simulink model "sim_qpOases_uncondensed"  (R2020b)
settings: Solver=FixedStepAuto  StartTime=0.0  StopTime=T_sim  FixedStep=dt  RelTol=1e-3
undefined symbols (not defined in the file): A_alpha1, A_init, A_TEC, Adyn_e, Adyn_t, b_alpha1, b_dyn, b_TEC, C, dt, H_e, H_t, L, lambda_beta, lb, m, N, NOISE, noise_bound_cl, nu, p, Sy_e, Sy_t, T_Track, T_Track2, T_Track3, ub, x0, y_T1, y_T2, y_T3, y_T4
libraries: simulink x5
settings Model: Creator=Fabian  LastModifiedBy=Fabian

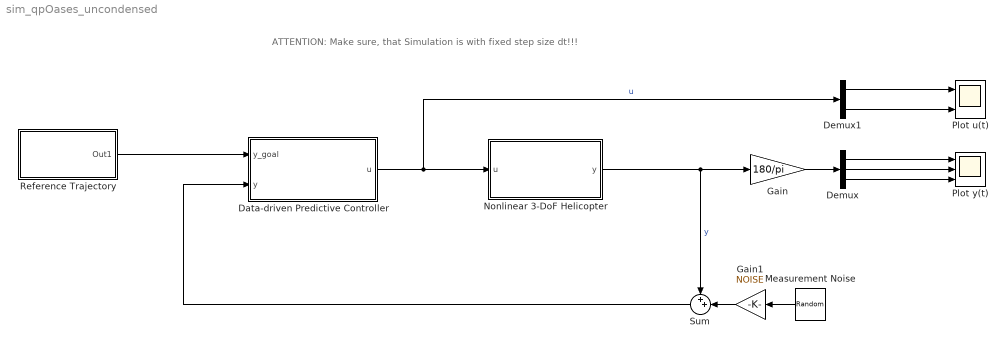
== system sim_qpOases_uncondensed ==
  note: ATTENTION: Make sure, that Simulation is with fixed step size dt!!!
  Data-driven Predictive Controller : Subsystem
  Demux : Demux  Outputs=3
  Demux1 : Demux  Outputs=2
  Gain : Gain  Gain=180/pi
  Gain1 : Gain  Gain=NOISE
  Measurement Noise : UniformRandomNumber  Minimum=-noise_bound_cl  Maximum=noise_bound_cl  Seed=[3;4;5]  SampleTime=dt
  Nonlinear 3-DoF Helicopter : Subsystem
  Plot u(t) : Scope  NumInputPorts=2
  Plot y(t) : Scope  NumInputPorts=3
  Reference Trajectory : Subsystem
  Sum : Sum  Inputs=++|
  wires:
  Data-driven Predictive Controller/1(u) -> Demux1/1, Nonlinear 3-DoF Helicopter/1(u)  "u"
  Measurement Noise/1 -> Gain1/1
  Nonlinear 3-DoF Helicopter/1(y) -> Gain/1, Sum/1  "y"
  Gain1/1 -> Sum/2
  Gain/1 -> Demux/1
  Sum/1 -> Data-driven Predictive Controller/2(y)
  Demux/2 -> Plot y(t)/2
  Demux/1 -> Plot y(t)/1
  Demux/3 -> Plot y(t)/3
  Reference Trajectory/1(Out1) -> Data-driven Predictive Controller/1(y_goal)
  Demux1/1 -> Plot u(t)/1
  Demux1/2 -> Plot u(t)/2

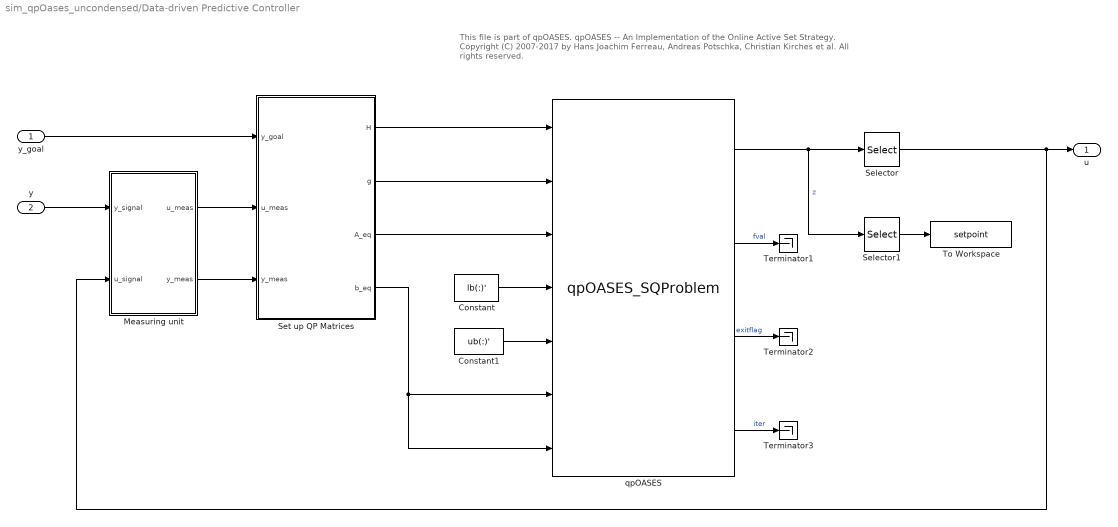
== system sim_qpOases_uncondensed/Data-driven Predictive Controller ==
  note: This file is part of qpOASES.
      |
      | qpOASES -- An Implementation of the Online Active Set Strategy.
      | Copyright (C) 2007-2017 by Hans Joachim Ferreau, Andreas Potschka, Christian Kirches et al.
      | All rights reserved.
  y_goal : Inport
  y : Inport  Port=2
  Constant : Constant  Value=lb(:)'
  Constant1 : Constant  Value=ub(:)'
  Measuring unit : Subsystem
  Selector : Selector  InputPortWidth=N-L+1+m*L+p*L+m+p+p*L+1  IndexOptions=Index vector (dialog)  Indices=N-L+1+m*nu+1:N-L+1+m*nu+m  OutputSizes=1
  Selector1 : Selector  InputPortWidth=N-L+1+m*L+p*L+m+p+p*L+1  IndexOptions=Index vector (dialog)  Indices=N-L+1+m*L+p*L+m+1:N-L+1+m*L+p*L+m+p  OutputSizes=1
  Set up QP Matrices : MATLAB Function  TreatAsAtomicUnit=on
  Terminator1 : Terminator
  Terminator2 : Terminator
  Terminator3 : Terminator
  To Workspace : ToWorkspace  VariableName=setpoint  SaveFormat=Timeseries  SampleTime=-1
  qpOASES : S-Function  FunctionName=qpOASES_SQProblem  SFunctionDeploymentMode=off  EnableBusSupport=off
  u : Outport
  wires:
  y/1 -> Measuring unit/1(y_signal)
  Measuring unit/1(u_meas) -> Set up QP Matrices/2(u_meas)
  Measuring unit/2(y_meas) -> Set up QP Matrices/3(y_meas)
  y_goal/1 -> Set up QP Matrices/1(y_goal)
  Selector/1 -> u/1, Measuring unit/2(u_signal)
  Set up QP Matrices/1(H) -> qpOASES/1
  qpOASES/1 -> Selector1/1, Selector/1  "z"
  Constant/1 -> qpOASES/4
  Set up QP Matrices/4(b_eq) -> qpOASES/6, qpOASES/7
  qpOASES/4 -> Terminator3/1  "iter"
  qpOASES/3 -> Terminator2/1  "exitflag"
  qpOASES/2 -> Terminator1/1  "fval"
  Set up QP Matrices/2(g) -> qpOASES/2
  Set up QP Matrices/3(A_eq) -> qpOASES/3
  Constant1/1 -> qpOASES/5
  Selector1/1 -> To Workspace/1

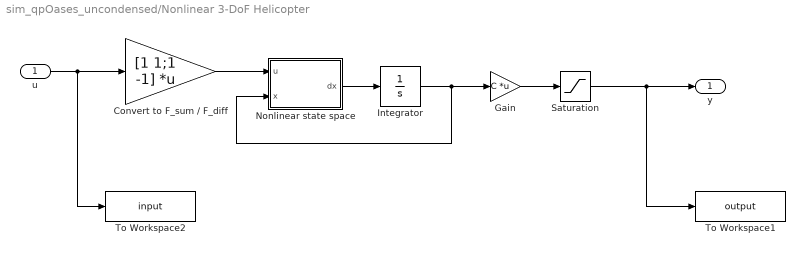
== system sim_qpOases_uncondensed/Nonlinear 3-DoF Helicopter ==
  u : Inport
  Convert to F_sum / F_diff : Gain  Gain=[1 1;1 -1]  Multiplication=Matrix(K*u)
  Gain : Gain  Gain=C  Multiplication=Matrix(K*u)
  Integrator : Integrator  InitialCondition=x0
  Nonlinear state space : MATLAB Function  TreatAsAtomicUnit=on
  Saturation : Saturate  UpperLimit=[inf; 33*pi/180; 90*pi/180]  LowerLimit=[-inf; -33*pi/180; -90*pi/180]
  To Workspace1 : ToWorkspace  VariableName=output  SaveFormat=Timeseries  SampleTime=-1
  To Workspace2 : ToWorkspace  VariableName=input  SaveFormat=Timeseries  SampleTime=-1
  y : Outport
  wires:
  Nonlinear state space/1(dx) -> Integrator/1
  Integrator/1 -> Nonlinear state space/2(x), Gain/1
  u/1 -> To Workspace2/1, Convert to F_sum / F_diff/1
  Convert to F_sum / F_diff/1 -> Nonlinear state space/1(u)
  Gain/1 -> Saturation/1
  Saturation/1 -> To Workspace1/1, y/1

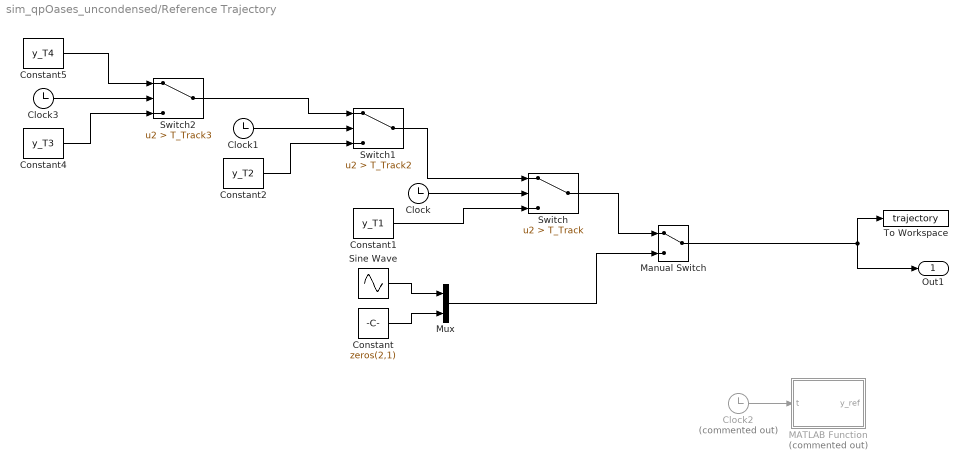
== system sim_qpOases_uncondensed/Reference Trajectory ==
  Clock : Clock
  Clock1 : Clock
  Clock2 : Clock  Commented=on
  Clock3 : Clock
  Constant : Constant  Value=zeros(2,1)
  Constant1 : Constant  Value=y_T1
  Constant2 : Constant  Value=y_T2
  Constant4 : Constant  Value=y_T3
  Constant5 : Constant  Value=y_T4
  MATLAB Function : MATLAB Function  Commented=on  TreatAsAtomicUnit=on
  Manual Switch : ManualSwitch
  Mux : Mux  Inputs=2
  Sine Wave : Sin  Amplitude=45*pi/180  Frequency=2*pi*1/25  Phase=-5*2*pi*1/25  SampleTime=0
  Switch : Switch  Criteria=u2 > Threshold  Threshold=T_Track
  Switch1 : Switch  Criteria=u2 > Threshold  Threshold=T_Track2
  Switch2 : Switch  Criteria=u2 > Threshold  Threshold=T_Track3
  To Workspace : ToWorkspace  VariableName=trajectory  SaveFormat=Timeseries  SampleTime=-1
  Out1 : Outport
  wires:
  Manual Switch/1 -> Out1/1, To Workspace/1
  Switch2/1 -> Switch1/1
  Mux/1 -> Manual Switch/2
  Constant2/1 -> Switch1/3
  Clock1/1 -> Switch1/2
  Clock/1 -> Switch/2
  Sine Wave/1 -> Mux/1
  Constant/1 -> Mux/2
  Switch/1 -> Manual Switch/1
  Switch1/1 -> Switch/1
  Constant1/1 -> Switch/3
  Clock2/1 -> MATLAB Function/1(t)
  Clock3/1 -> Switch2/2
  Constant5/1 -> Switch2/1
  Constant4/1 -> Switch2/3

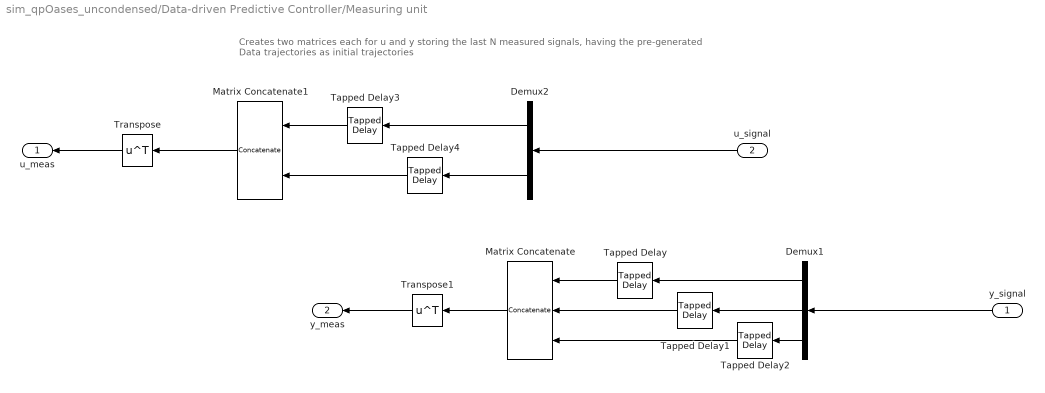
== system sim_qpOases_uncondensed/Data-driven Predictive Controller/Measuring unit ==
  note: Creates two matrices each for u and y storing the last N measured signals,
      | having the pre-generated Data trajectories as initial trajectories
  y_signal : Inport
  u_signal : Inport  Port=2
  Demux1 : Demux  Outputs=3
  Demux2 : Demux  Outputs=2
  Matrix Concatenate : Concatenate  NumInputs=3  Mode=Multidimensional array  ConcatenateDimension=2
  Matrix Concatenate1 : Concatenate  Mode=Multidimensional array  ConcatenateDimension=2
  Tapped Delay : simulink/Discrete/Tapped Delay  vinit=x0(1)*ones(nu,1)  samptime=-1  NumDelays=nu  DelayOrder=Oldest  includeCurrent=off
  Tapped Delay1 : simulink/Discrete/Tapped Delay  vinit=x0(3)*ones(nu,1)  samptime=-1  NumDelays=nu  DelayOrder=Oldest  includeCurrent=off
  Tapped Delay2 : simulink/Discrete/Tapped Delay  vinit=x0(5)*ones(nu,1)  samptime=-1  NumDelays=nu  DelayOrder=Oldest  includeCurrent=off
  Tapped Delay3 : simulink/Discrete/Tapped Delay  vinit=0  samptime=-1  NumDelays=nu  DelayOrder=Oldest  includeCurrent=off
  Tapped Delay4 : simulink/Discrete/Tapped Delay  vinit=0  samptime=-1  NumDelays=nu  DelayOrder=Oldest  includeCurrent=off
  Transpose : Math  Operator=transpose  SaturateOnIntegerOverflow=on
  Transpose1 : Math  Operator=transpose  SaturateOnIntegerOverflow=on
  u_meas : Outport
  y_meas : Outport  Port=2
  wires:
  Demux2/2 -> Tapped Delay4/1
  Demux2/1 -> Tapped Delay3/1
  Tapped Delay3/1 -> Matrix Concatenate1/1
  Demux1/1 -> Tapped Delay/1
  Demux1/2 -> Tapped Delay1/1
  Tapped Delay4/1 -> Matrix Concatenate1/2
  Demux1/3 -> Tapped Delay2/1
  Tapped Delay1/1 -> Matrix Concatenate/2
  Tapped Delay/1 -> Matrix Concatenate/1
  Tapped Delay2/1 -> Matrix Concatenate/3
  u_signal/1 -> Demux2/1
  y_signal/1 -> Demux1/1
  Matrix Concatenate1/1 -> Transpose/1
  Transpose/1 -> u_meas/1
  Matrix Concatenate/1 -> Transpose1/1
  Transpose1/1 -> y_meas/1

== matlab function sim_qpOases_uncondensed/Reference Trajectory/MATLAB Function ==
  data: t input; y_ref output
function y_ref = fcn(t)
       

    y_home_v = [0*pi/180; 0*pi/180; 0];  
    y_cargo_v = [90*pi/180; 0*pi/180; 0]; 
    y_cargo = [90*pi/180; -22*pi/180; 0];
    y_drop_v = [450*pi/180; 0*pi/180; 0];
    y_drop = [450*pi/180; -22*pi/180; 0];
    y_home = [0*pi/180; -27*pi/180; 0];

    if (0 <= t) && t < 5
        y_ref = y_home_v;
    elseif (5 <= t) && t < 17
        y_ref = y_cargo_v;
    elseif (17 <= t) && t < 30
        y_ref = y_cargo;
    elseif (30 <= t) && t < 35
        y_ref = y_cargo_v;
    elseif (35 <= t) && t < 50
        y_ref = y_drop_v;
    elseif (50 <= t) && t < 65
        y_ref = y_drop;
    elseif (65 <= t) && t < 70
        y_ref = y_drop_v;
    elseif (70 <= t) && t < 90
        y_ref = y_home_v;
    elseif t > 90
        y_ref = y_home;
    else
        y_ref = y_home;
    end

end

== matlab function sim_qpOases_uncondensed/Nonlinear 3-DoF Helicopter/Nonlinear state space ==
  data: u input; x input; dx output
function dx = fcn(u,x)

%%%%%%%%%%%%%%%%%%%%%%%%%%%%%%%%%%%%%%%%%%%%%%%%%%%%%%%%%%%%%%%%%%%%%%%%
%%%%%%%%%%%%%%%%%%%%% ATTENTION %%%%%%%%%%%%%%%%%%%%%%%%%%%%%%%%%%%%%%%%
%%%% Input is F_sum and F_diff, not F_front and F_back !! %%%%%%%%%%%%%%
%%%%%%%%%%%%%%%%%%%%%%%%%%%%%%%%%%%%%%%%%%%%%%%%%%%%%%%%%%%%%%%%%%%%%%%%

    m_H = 1.322;
    m_A = 2.638;

    Jxx = 1.1455;
    Jyy = 1.1184;
    Jzz = 0.032;

    r = 0.1775;

    rHx = -0.089;
    rHz = 0.655;
    rAHx = -0.034;
    rAHz = 0.0193;

    g = 9.81;
    
    dalph = x(2);
    bet = x(3);
    dbet = x(4);
    gam = x(5);
    dgam = x(6);
    
    Fsum = u(1);
    Fdiff = u(2);
    
    dx = [dalph;...
     1/Jxx * Fsum*sin(gam) * (rHx*sin(bet) - rHz*cos(bet));...
     dbet;...
     1/Jyy * (-(m_A+m_H)*g *(rAHz*cos(bet) - rAHx*sin(bet)) + Fsum * rHz*cos(gam));...
     dgam;...
     -1/Jzz * r * Fdiff];

end

== matlab function sim_qpOases_uncondensed/Data-driven Predictive Controller/Set up QP Matrices ==
  data: y_goal input; u_meas input; H output; y_meas input; g output size=[1, N-L+1 + (m+p)*L + m+p + p*L + 1]; b_dyn parameter; A_init parameter; b_TEC parameter; b_alpha1 parameter; A_TEC parameter; A_alpha1 parameter; m parameter; p parameter; N parameter; L parameter; lambda_beta parameter; A_eq output; b_eq output; H_t parameter; H_e parameter; Adyn_t parameter; Adyn_e parameter; Sy_t parameter; Sy_e parameter
function [H, g, A_eq, b_eq] = qpSetup(y_goal, u_meas, y_meas, b_dyn, A_init, b_TEC, b_alpha1, A_TEC, A_alpha1, m, p, N, L, lambda_beta, H_t, H_e, Adyn_t, Adyn_e, Sy_t, Sy_e)
    
    % ATTENTION: Simulation Step Size must be dt (fixed)!!!

    %% Update Init Data
    
    % Take past nu measurements for init
    u_init = u_meas(:);
    y_init = y_meas(:);
        
    b_init = [u_init(:); y_init(:)];
    
    %% Schedule data
    
    travel = 1;
    if y_goal(2) < 0
        travel = 0;
    end
    
    if travel
        % Travel taks, use respective data and parameters
        
        H = H_t(:)';
        
        % Include tracking point y_goal
        g = zeros(1,710);
        g(1, N-L+1+(m+p)*L+m+1 : N-L+1+(m+p)*L+m+p) = -2*(Sy_t*y_goal)';
        %g = [zeros(N-L+1,1);zeros((m+p)*L+m,1);-2*Sy_t*y_goal;zeros(p*L,1);-lambda_beta];
        
        Aeq = [Adyn_t; A_init; A_TEC; A_alpha1];
        A_eq = Aeq(:)';
        beq = [b_dyn ; b_init; b_TEC; b_alpha1];
        b_eq = beq(:)';

    else
        % Elevation taks, use respective data and parameters
        
        H = H_e(:)';
        
        % Include tracking point y_goal
        g = zeros(1,710);
        g(1, N-L+1+(m+p)*L+m+1 : N-L+1+(m+p)*L+m+p) = -2*(Sy_e*y_goal)';
        %g = [zeros(N-L+1,1);zeros((m+p)*L+m,1);-2*Sy_e*y_goal;zeros(p*L,1);-lambda_beta];
        
        Aeq = [Adyn_e; A_init; A_TEC; A_alpha1];
        A_eq = Aeq(:)';
        beq = [b_dyn ; b_init; b_TEC; b_alpha1];
        b_eq = beq(:)';

    end
    
end
